simulink model "t7_videoclase2_masa_resorte_amortiguador"  (R2022b)
settings: Solver=ode4  StartTime=0.0  StopTime=50  FixedStep=0.01  MaxStep=1.0  RelTol=1e-3
model workspace (MAT data in the model file):
  c = 1
  k = 2
  m = 3
settings Model: Creator=jibmo  LastModifiedBy=scpmoxxa
settings DataIOCC: SaveFormat=Array  SaveState=on

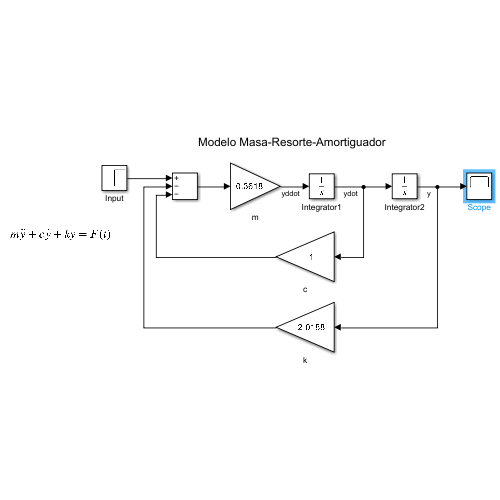
[thumbnail: Simulink's stored preview of the top-level diagram]
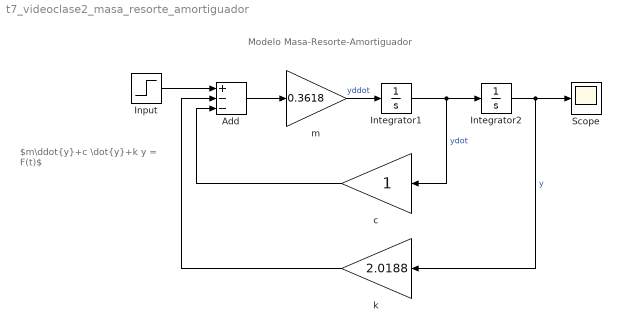
== system t7_videoclase2_masa_resorte_amortiguador ==
  note: Modelo Masa-Resorte-Amortiguador
  note: $m\ddot{y}+c \dot{y}+k y = F(t)$
  Add : Sum  Inputs=+--
  Input : Step  SampleTime=0
  Integrator1 : Integrator
  Integrator2 : Integrator
  Scope : Scope
  c : Gain  SCDEnableBlockLinearizationSpecification=on
  k : Gain  SCDEnableBlockLinearizationSpecification=on  Gain=2.0188
  m : Gain  SCDEnableBlockLinearizationSpecification=on  Gain=0.3618
  wires:
  m/1 -> Integrator1/1  "yddot"
  Integrator1/1 -> c/1, Integrator2/1  "ydot"
  Integrator2/1 -> k/1, Scope/1  "y"
  Add/1 -> m/1
  c/1 -> Add/3
  k/1 -> Add/2
  Input/1 -> Add/1
